simulink model "Dac_tinh_dong_co_KDB_roto_dayQuan"  (R2019a)
settings: Solver=VariableStepAuto  StartTime=0.0  StopTime=1  RelTol=1e-3
libraries: powerlib x14, simulink x1
settings Model: Creator=Admin  LastModifiedBy=Admin

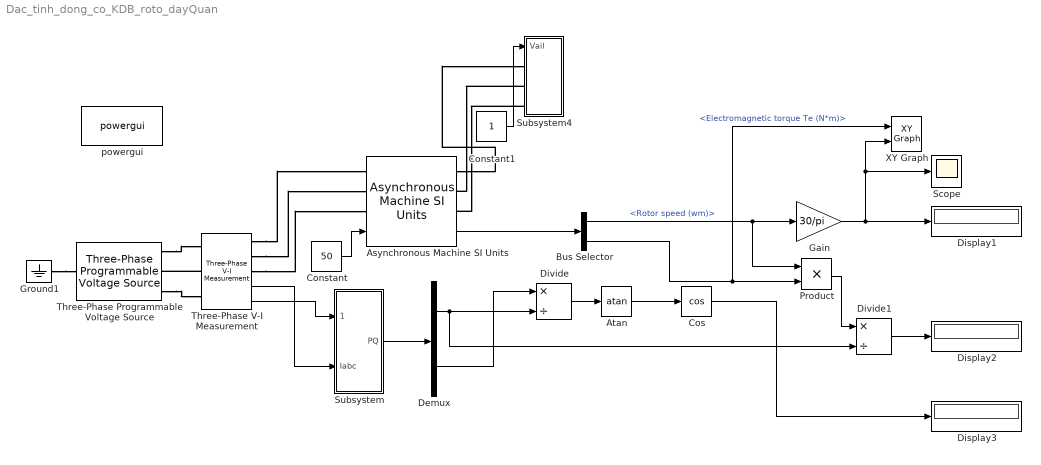
== system Dac_tinh_dong_co_KDB_roto_dayQuan ==
  Asynchronous Machine SI Units : powerlib/Machines/Asynchronous Machine SI Units  RotorType=Wound  PresetModel=No  MechanicalLoad=Torque Tm  ShowDetailedParameters=on  ReferenceFrame=Rotor  Units=SI  MeasurementBus=off  NominalParameters=[3.3667 220 50]  Stator=[0.431 0.00246]  Rotor=[0.579 0.00315]  Cage1=[0.4155 0.002066]  Cage2=[0.4168 0.0003495]  Lm=0.101  Mechanical=[0.1 0 4]  PolePairs=2  InitialConditions=[0 0 0 0 0 0 0 0]  SimulateSaturation=off  Saturation=[14.03593122, 27.81365428, 53.79336849, 72.68890987, 97.98006896, 148.6815601, 215.7428561, 302.9841135, 428.7778367 ; 230, 322, 414, 460, 506, 552, 598, 644, 690]  LoadFlowParameters=1492000  TsPowergui=0  TsBlock=-1  IterativeModel=Trapezoidal non iterative  IterativeDiscreteModel=Trapezoidal non iterative  Pmec=1.492e+006
      settings: SourceProductName=Simscape Electrical
  Atan : Trigonometry  Operator=atan
  Bus Selector : BusSelector  OutputSignals=Mechanical.Rotor speed (wm),Mechanical.Electromagnetic torque Te (N*m)
  Constant : Constant  Value=50
  Constant1 : Constant
  Cos : Trigonometry  Operator=cos
  Demux : Demux  Outputs=2
  Display1 : Display
  Display2 : Display
  Display3 : Display
  Divide : Product  Inputs=*/
  Divide1 : Product  Inputs=*/
  Gain : Gain  Gain=30/pi
  Ground1 : powerlib/Elements/Ground  LConnTagsString=a
      settings: SourceProductName=Simscape Electrical
  Product : Product
  Scope : Scope
  Subsystem : Subsystem
  Subsystem4 : Subsystem
  Three-Phase Programmable Voltage Source : powerlib/Electrical Sources/Three-Phase Programmable Voltage Source  PositiveSequence="[220  0 50]"  VariationEntity=None  VariationType=Table of time-amplitude pairs  VariationTypeAlt=Step  VariationStep=0.5  VariationRate=10  VariationMagnitude=0.3  VariationFrequency=2  VariationTiming=[1 2]  VariationPhaseA=off  Amplitudes=[1 0.8 1.2 1.0]  TimeValues=[0 0.1 0.15 0.2]  HarmonicGeneration=off  HarmonicA=[3 0.2 -25 0]  HarmonicB=[2 0.15 35 2]  Timing="[0.05  3]"  BusType=swing  Pref=0  Qref=0  Qmin=-inf  Qmax=inf
      settings: SourceProductName=Simscape Electrical
  Three-Phase V-I Measurement : powerlib/Measurements/Three-Phase V-I Measurement  VoltageMeasurement=phase-to-ground  SetLabelV=off  LabelV=Vabc  Vpu=off  VpuLL=off  CurrentMeasurement=yes  SetLabelI=off  LabelI=Iabc  Ipu=off  Pbase=100e6  Vbase=500e3  OutputType=Complex  PhasorSimulation=off  PSBequivalent=0
      settings: SourceProductName=Simscape Electrical
  XY Graph : simulink/Sinks/XY Graph  xmin=0  xmax=1500  ymin=0  ymax=500  st=1
  powergui : powerlib/powergui  Priority=1  SimulationMode=Continuous  SampleTime=50e-6  frequency=60  Iterations=50  frequencyindice=50  Pbase=100e6  ErrMax=1e-4  UnitsV=kV  UnitsW=MW  buscounter=0  FunctionMessages=off  echomessages=off  EnableUseOfTLC=off  CurrentSourceSwitches=off  DisableSnubberDevices=off  DisableRonSwitches=off  DisableVfSwitches=off  DisplayEquations=off  AutomaticDiscreteSolvers=off  SolverType=Tustin/Backward Euler (TBE)  Interpol=off  ExternalGateDelay=off  methode=off  Ts=100  x0status=blocks  SPID=on  SwTol=0  HookPort=off  NonlinearTolerance=0  nMaxIteration=15  ContinueOnMaxIteration=off  RestoreLinks=warning  ResistiveCurrentMeasurement=off  Frange=[0:2:500]  Ylog=off  Xlog=on  ShowGrid=off  save=off  variable=ZData  structure=0  ZoomFFT=off  StartTime=0.0  cycles=1  DisplayStyle=1  fundamental=60  FreqAxis=off  MaxFrequency=1000  frequencyindicesteady=1  RmsSteady=1  display=off
      settings: SourceProductName=Simscape Electrical
  wires:
  Constant/1 -> Asynchronous Machine SI Units/1
  Demux/1 -> Divide1/2, Divide/2
  Demux/2 -> Divide/1
  Divide/1 -> Atan/1
  Atan/1 -> Cos/1
  Asynchronous Machine SI Units/1 -> Bus Selector/1
  Bus Selector/1 -> Product/1, Gain/1  "<Rotor speed (wm)>"
  Bus Selector/2 -> XY Graph/1, Product/2  "<Electromagnetic torque Te (N*m)>"
  Product/1 -> Divide1/1
  Subsystem/1("PQ ") -> Demux/1
  Constant1/1 -> Subsystem4/1("Vail ")
  Three-Phase V-I Measurement/2 -> Subsystem/2("Iabc ")
  Three-Phase V-I Measurement/1 -> Subsystem/1("Vacc ")
  Cos/1 -> Display3/1
  Divide1/1 -> Display2/1
  Gain/1 -> Scope/1, XY Graph/2, Display1/1
  connections:
  Three-Phase V-I Measurement/RConn3 -- Asynchronous Machine SI Units/LConn3
  Three-Phase V-I Measurement/RConn2 -- Asynchronous Machine SI Units/LConn2
  Three-Phase V-I Measurement/RConn1 -- Asynchronous Machine SI Units/LConn1
  Ground1/LConn1 -- Three-Phase Programmable Voltage Source/LConn1
  Asynchronous Machine SI Units/RConn3 -- Subsystem4/LConn1
  Subsystem4/LConn2 -- Asynchronous Machine SI Units/RConn2
  Subsystem4/LConn3 -- Asynchronous Machine SI Units/RConn1
  Three-Phase Programmable Voltage Source/RConn3 -- Three-Phase V-I Measurement/LConn3
  Three-Phase V-I Measurement/LConn2 -- Three-Phase Programmable Voltage Source/RConn2
  Three-Phase Programmable Voltage Source/RConn1 -- Three-Phase V-I Measurement/LConn1

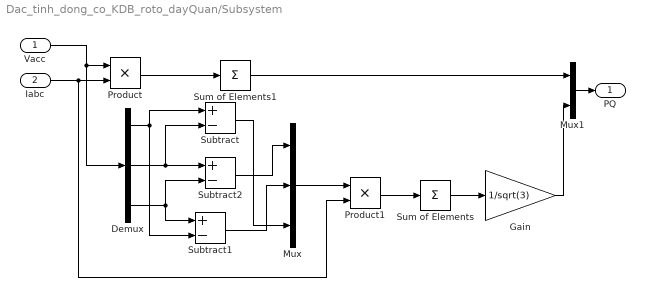
== system Dac_tinh_dong_co_KDB_roto_dayQuan/Subsystem ==
  "Vacc " : Inport
  "Iabc " : Inport  Port=2
  Demux : Demux  Outputs=3
  Gain : Gain  Gain=1/sqrt(3)
  Mux : Mux  Inputs=3
  Mux1 : Mux  Inputs=2
  Product : Product
  Product1 : Product
  Subtract : Sum  Inputs=+-
  Subtract1 : Sum  Inputs=+-
  Subtract2 : Sum  Inputs=+-
  Sum of Elements : Sum  Inputs=+
  Sum of Elements1 : Sum  Inputs=+
  "PQ " : Outport
  wires:
  Demux/1 -> Subtract1/2, Subtract/1
  Product/1 -> Sum of Elements1/1
  Demux/2 -> Subtract2/1, Subtract/2
  Gain/1 -> Mux1/2
  Subtract/1 -> Mux/3
  Subtract2/1 -> Mux/1
  Sum of Elements1/1 -> Mux1/1
  Demux/3 -> Subtract1/1, Subtract2/2
  Product1/1 -> Sum of Elements/1
  Mux1/1 -> "PQ "/1
  Sum of Elements/1 -> Gain/1
  "Vacc "/1 -> Demux/1, Product/1
  Subtract1/1 -> Mux/2
  Mux/1 -> Product1/1
  "Iabc "/1 -> Product1/2, Product/2

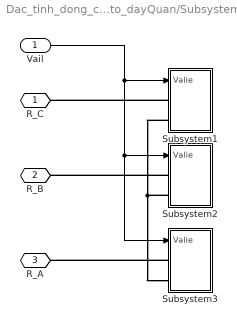
== system Dac_tinh_dong_co_KDB_roto_dayQuan/Subsystem4 ==
  "Vail " : Inport
  Subsystem1 : Subsystem
  Subsystem2 : Subsystem
  Subsystem3 : Subsystem
  R_C : PMIOPort  Side=Left
  R_B : PMIOPort  Port=2  Side=Left
  R_A : PMIOPort  Port=3  Side=Left
  wires:
  "Vail "/1 -> Subsystem3/1(Valie), Subsystem2/1(Valie), Subsystem1/1(Valie)
  connections:
  Subsystem2/LConn1 -- R_B/RConn1
  Subsystem1/LConn1 -- R_C/RConn1
  Subsystem3/LConn1 -- R_A/RConn1
  Subsystem1/LConn2 -- Subsystem2/LConn2 -- Subsystem3/LConn2

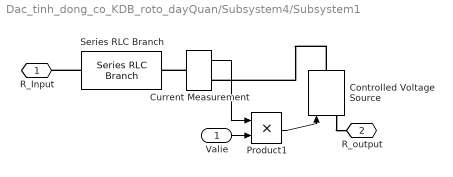
== system Dac_tinh_dong_co_KDB_roto_dayQuan/Subsystem4/Subsystem1 ==
  Valie : Inport
  Controlled Voltage Source : powerlib/Electrical Sources/Controlled Voltage Source  Initialize=on  Source_Type=DC  Amplitude=0  Phase=0  Frequency=0  Measurements=None
      settings: SourceProductName=Simscape Electrical
  Current Measurement : powerlib/Measurements/Current Measurement  PhasorSimulation=off  OutputType=Complex  PSBequivalent=0
      settings: SourceProductName=Simscape Electrical
  Product1 : Product
  Series RLC Branch : powerlib/Elements/Series RLC Branch  LConnTagsString=__new0  RConnTagsString=__new0  BranchType=R  Resistance=0.001  Inductance=0  SetiL0=off  InitialCurrent=0  Capacitance=1000000000  Setx0=off  InitialVoltage=0  Measurements=None
      settings: SourceProductName=Simscape Electrical
  R_Input : PMIOPort  Side=Left
  R_output : PMIOPort  Port=2  Side=Left
  wires:
  Product1/1 -> Controlled Voltage Source/1
  Current Measurement/1 -> Product1/1
  Valie/1 -> Product1/2
  connections:
  Controlled Voltage Source/RConn1 -- Current Measurement/RConn1
  Current Measurement/LConn1 -- Series RLC Branch/RConn1
  Controlled Voltage Source/LConn1 -- R_output/RConn1
  Series RLC Branch/LConn1 -- R_Input/RConn1

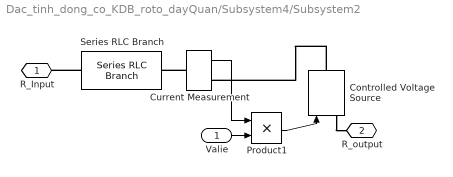
== system Dac_tinh_dong_co_KDB_roto_dayQuan/Subsystem4/Subsystem2 ==
  Valie : Inport
  Controlled Voltage Source : powerlib/Electrical Sources/Controlled Voltage Source  Initialize=on  Source_Type=DC  Amplitude=0  Phase=0  Frequency=0  Measurements=None
      settings: SourceProductName=Simscape Electrical
  Current Measurement : powerlib/Measurements/Current Measurement  PhasorSimulation=off  OutputType=Complex  PSBequivalent=0
      settings: SourceProductName=Simscape Electrical
  Product1 : Product
  Series RLC Branch : powerlib/Elements/Series RLC Branch  LConnTagsString=__new0  RConnTagsString=__new0  BranchType=R  Resistance=0.001  Inductance=0  SetiL0=off  InitialCurrent=0  Capacitance=1000000000  Setx0=off  InitialVoltage=0  Measurements=None
      settings: SourceProductName=Simscape Electrical
  R_Input : PMIOPort  Side=Left
  R_output : PMIOPort  Port=2  Side=Left
  wires:
  Product1/1 -> Controlled Voltage Source/1
  Current Measurement/1 -> Product1/1
  Valie/1 -> Product1/2
  connections:
  Controlled Voltage Source/RConn1 -- Current Measurement/RConn1
  Current Measurement/LConn1 -- Series RLC Branch/RConn1
  Controlled Voltage Source/LConn1 -- R_output/RConn1
  Series RLC Branch/LConn1 -- R_Input/RConn1

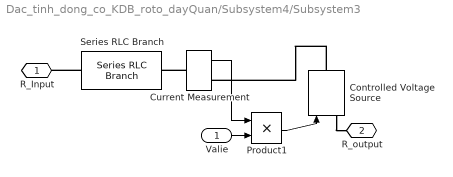
== system Dac_tinh_dong_co_KDB_roto_dayQuan/Subsystem4/Subsystem3 ==
  Valie : Inport
  Controlled Voltage Source : powerlib/Electrical Sources/Controlled Voltage Source  Initialize=on  Source_Type=DC  Amplitude=0  Phase=0  Frequency=0  Measurements=None
      settings: SourceProductName=Simscape Electrical
  Current Measurement : powerlib/Measurements/Current Measurement  PhasorSimulation=off  OutputType=Complex  PSBequivalent=0
      settings: SourceProductName=Simscape Electrical
  Product1 : Product
  Series RLC Branch : powerlib/Elements/Series RLC Branch  LConnTagsString=__new0  RConnTagsString=__new0  BranchType=R  Resistance=0.001  Inductance=0  SetiL0=off  InitialCurrent=0  Capacitance=1000000000  Setx0=off  InitialVoltage=0  Measurements=None
      settings: SourceProductName=Simscape Electrical
  R_Input : PMIOPort  Side=Left
  R_output : PMIOPort  Port=2  Side=Left
  wires:
  Product1/1 -> Controlled Voltage Source/1
  Current Measurement/1 -> Product1/1
  Valie/1 -> Product1/2
  connections:
  Controlled Voltage Source/RConn1 -- Current Measurement/RConn1
  Current Measurement/LConn1 -- Series RLC Branch/RConn1
  Controlled Voltage Source/LConn1 -- R_output/RConn1
  Series RLC Branch/LConn1 -- R_Input/RConn1
